simulink model "Qmod"
settings: Solver=ode45  StartTime=0.0  StopTime=10.0  RelTol=1e-3
values from neighbouring files (symbols this model uses):
  g = 9.81    [Qconst.m]
  Ixx = 1    [Qconst.m]
  Iyy = 1    [Qconst.m]
  Izz = 1    [Qconst.m]
  k = 1    [Qconst.m]
  m = 1    [Qconst.m]
settings Model: Creator=DNI 38876767  LastModifiedBy=gabriel
settings DataIOCC: LimitDataPoints=on  SaveFormat=Array  ReturnWorkspaceOutputs=off
settings OptimizationCC: ExpressionDepthLimit=2147483647  LifeSpan=inf  SimCompilerOptimization=Off
settings DebuggingCC: UnderspecifiedInitializationDetection=Classic  MergeDetectMultiDrivingBlocksExec=none  SolverPrmCheckMsg=warning  MultiTaskDSMMsg=warning  MultiTaskCondExecSysMsg=none  FcnCallInpInsideContextMsg=Enable All  FrameProcessingCompatibilityMsg=warning  StateNameClashWarn=warning  StrictBusMsg=None  SFUnexpectedBacktrackingDiag=warning  SFNoUnconditionalDefaultTransitionDiag=warning
settings HardwareCC: ProdBitPerPointer=32  ProdLargestAtomicFloat=None  ProdIntDivRoundTo=Undefined  ProdEndianess=Unspecified  ProdWordSize=32  ProdHWDeviceType=32-bit Generic
settings ModelReferenceCC: PropagateSignalLabelsOutOfModel=off
settings SFSimCC: SimUseLocalCustomCode=off
settings RTWCC: RTWUseLocalCustomCode=off  IncludeERTFirstTime=on  RTWCompilerOptimization=Off
settings CodeAppCC: CustomSymbolStrType=$N$R$M
settings GRTTargetCC: CodeReplacementLibrary=ANSI_C  GeneratePreprocessorConditionals=Disable all  CPPClassGenCompliant=off

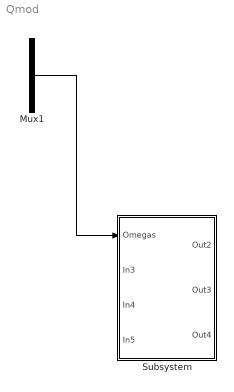
== system Qmod ==
  Mux1 : Mux
  Subsystem : Subsystem
  wires:
  Mux1/1 -> Subsystem/1("Omegas ")

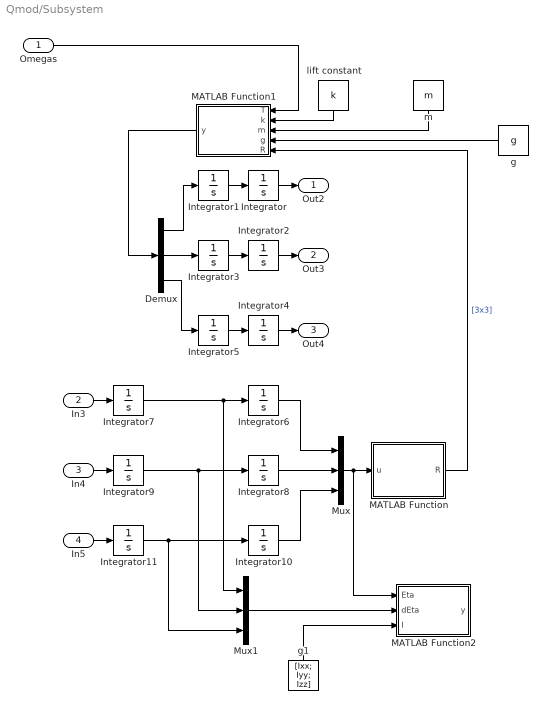
== system Qmod/Subsystem ==
  "Omegas " : Inport
  In3 : Inport  Port=2
  In4 : Inport  Port=3
  In5 : Inport  Port=4
  Demux : Demux  Outputs=3
  Integrator{,2..11} (11 alike) : Integrator
  Integrator1 : Integrator  InitialCondition=1
  MATLAB Function : MATLAB Function  TreatAsAtomicUnit=on
  MATLAB Function1 : MATLAB Function  TreatAsAtomicUnit=on
  MATLAB Function2 : MATLAB Function  TreatAsAtomicUnit=on
  Mux : Mux  Inputs=3
  Mux1 : Mux  Inputs=3
  g : Constant  Value=g
  g1 : Constant  Value=[Ixx; Iyy; Izz]
  lift constant : Constant  Value=k
  m : Constant  Value=m
  Out2 : Outport
  Out3 : Outport  Port=2
  Out4 : Outport  Port=3
  wires:
  Integrator9/1 -> Integrator8/1, Mux1/2
  MATLAB Function1/1(y) -> Demux/1
  Integrator11/1 -> Integrator10/1, Mux1/3
  Integrator5/1 -> Integrator4/1
  Integrator7/1 -> Integrator6/1, Mux1/1
  Integrator3/1 -> Integrator2/1
  Integrator/1 -> Out2/1
  In3/1 -> Integrator7/1
  MATLAB Function/1(R) -> MATLAB Function1/5(R)  "[3x3]"
  Integrator4/1 -> Out4/1
  In5/1 -> Integrator11/1
  Integrator2/1 -> Out3/1
  In4/1 -> Integrator9/1
  "Omegas "/1 -> MATLAB Function1/1(T)
  Demux/3 -> Integrator5/1
  Integrator8/1 -> Mux/2
  Mux/1 -> MATLAB Function/1(u), MATLAB Function2/1(Eta)
  Demux/1 -> Integrator1/1
  Demux/2 -> Integrator3/1
  Integrator1/1 -> Integrator/1
  Integrator10/1 -> Mux/3
  Integrator6/1 -> Mux/1
  lift constant/1 -> MATLAB Function1/2(k)
  m/1 -> MATLAB Function1/3(m)
  g/1 -> MATLAB Function1/4(g)
  Mux1/1 -> MATLAB Function2/2(dEta)
  g1/1 -> MATLAB Function2/3(I)

== matlab function Qmod/Subsystem/MATLAB Function1 ==
  data: T input; k input; m input; g input; y output; R input
function y = fcn(T,k,m,g,R)
%#codegen
%k=1;
%eml.extrinsic('k');
Thrust=[0; 0; k*(T(1)+T(2)+T(3)+T(4))/m];
%y = R*Thrust;
y=R*Thrust-[0; 0; -g];

== matlab function Qmod/Subsystem/MATLAB Function ==
  data: u input; R output
function R = fcn(u)
%#codegen
%H=sym('H')
Phi=u(1);
Theta=u(2);
Psi=u(3);

R = [[cos(Psi)*cos(Theta) cos(Psi)*sin(Theta)*sin(Phi)-sin(Psi)*cos(Phi) cos(Psi)*sin(Theta)*cos(Phi)+sin(Psi)*sin(Phi)];
     [sin(Psi)*cos(Theta) sin(Psi)*sin(Theta)*sin(Phi)+cos(Psi)*cos(Phi) sin(Psi)*sin(Theta)*cos(Phi)-cos(Psi)*sin(Phi)];
     [-sin(Theta) cos(Theta)*sin(Phi) cos(Theta)*cos(Phi)]];

== matlab function Qmod/Subsystem/MATLAB Function2 ==
  data: Eta input; y output; dEta input; I input
function y = fcn(Eta,dEta,I)
%#codegen

Phi=Eta(1);
Theta=Eta(2);
Psi=Eta(3);

dPhi=dEta(1);
dTheta=dEta(2);
dPsi=dEta(3);

Ixx=I(1);
Iyy=I(2);
Izz=I(3);

C11=;
C12=;
C13=;

C21=;
C22=;
C23=;

C31=;
C32=;
C33=;

C=[[C11 C12 C13];
   [C21 C22 C23];
   [C31 C32 C33]];
y = 1;
